simulink model "WorstCaseInertia"  (R2020a)
settings: Solver=VariableStepAuto  StartTime=0.0  StopTime=inf  RelTol=1e-3
libraries: vrlib x7, aerolibanimutils x1, RobotG18_Blocos x1
settings Model: Creator=Catarina  LastModifiedBy=Catarina

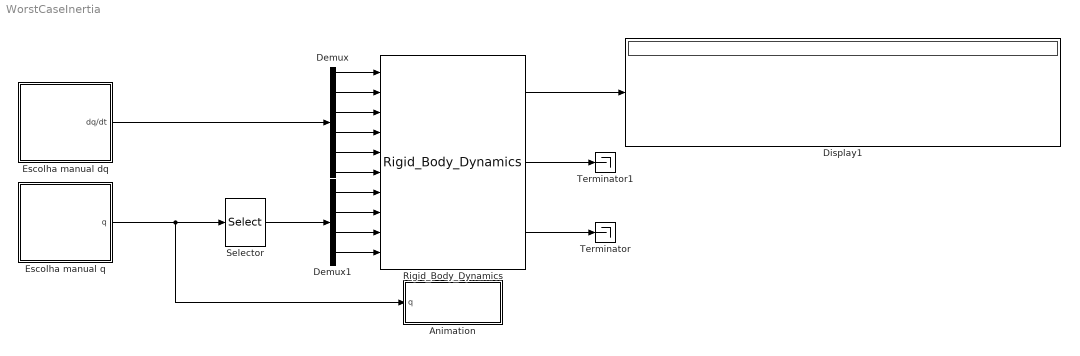
== system WorstCaseInertia ==
  "Animation " : Subsystem
  Demux : Demux  Outputs=6
  Demux1 : Demux
  Display1 : Display
  Escolha manual dq : Subsystem  mask{q1=9.800, q2=-1.400, q3=10.0, q4=-10.0, q5=-5.600, q6=-6.400}
      mask prompts: q1 "dq1"; q2 "dq2"; q3 "dq3"; q4 "dq4"; q5 "dq5"; q6 "dq6"
  "Escolha manual q " : Subsystem  mask{q1=0, q2=0, q3=0, q4=-111, q5=-90.0, q6=0}
  Rigid_Body_Dynamics : RobotG18_Blocos/Rigid_Body_Dynamics  SystemSampleTime=-1  Latency=0  AutoFrameSizeCalculation=off
  Selector : Selector  InputPortWidth=6  IndexOptions=Index vector (dialog)  Indices=[2 3 4 5]  OutputSizes=1
  Terminator : Terminator
  Terminator1 : Terminator
  wires:
  Demux/6 -> Rigid_Body_Dynamics/6
  Demux1/1 -> Rigid_Body_Dynamics/7
  Demux/3 -> Rigid_Body_Dynamics/3
  Demux/5 -> Rigid_Body_Dynamics/5
  Demux/4 -> Rigid_Body_Dynamics/4
  Demux1/2 -> Rigid_Body_Dynamics/8
  Demux/1 -> Rigid_Body_Dynamics/1
  Demux1/3 -> Rigid_Body_Dynamics/9
  Demux1/4 -> Rigid_Body_Dynamics/10
  Demux/2 -> Rigid_Body_Dynamics/2
  "Escolha manual q "/1("q ") -> "Animation "/1("q "), Selector/1
  Escolha manual dq/1("dq/dt ") -> Demux/1
  Selector/1 -> Demux1/1
  Rigid_Body_Dynamics/2 -> Terminator1/1
  Rigid_Body_Dynamics/3 -> Terminator/1
  Rigid_Body_Dynamics/1 -> Display1/1

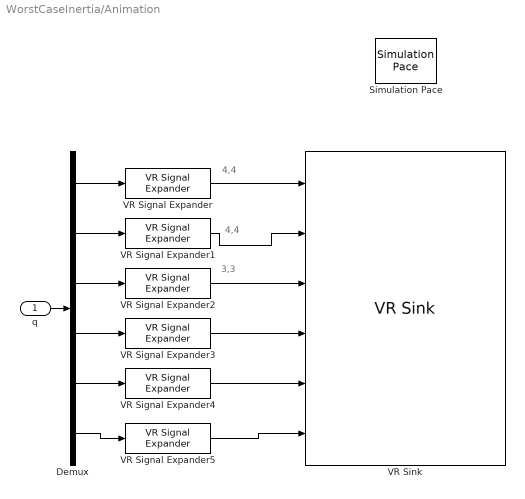
== system WorstCaseInertia/Animation  ==
  note: 4,4
  note: 3,3
  note: 4,4
  "q " : Inport
  Demux : Demux  Outputs=6
  Simulation Pace : aerolibanimutils/Simulation Pace  SimulationPace=1  SleepMode=Auto  OutputPaceError=off  SampleTime=1/30
  VR Signal Expander{,1..5} (6 alike) : vrlib/VR Signal Expander  outwidth=4  outidx=4
  VR Sink : vrlib/VR Sink  InstantiateOnLoad=on  SampleTime=1/30  ViewEnable=on  RemoteChange=off  RemoteView=off  FieldsWritten=Jt1_DH_dv.rotation.4.1.1.double#Jt2_DH_dv.rotation.4.1.1.double#Jt3_DH_dv.rotation.4.1.1.double#Jt4_DH_dv.rotation.4.1.1.double#Jt5_DH_dv.rotation.4.1.1.double#Jt6_DH_dv.rotation.4.1.1.double  WorldFileName=RobotG18_Opt_NoAxes.wrl  WorldDescription=D-H Reference Frames for Virtual Reality Robot  AutoView=off  VideoDimensions=[]  AllowVariableSize=off  FigureProperties="{'Position', 'Name', 'Viewpoint', 'CameraBound', 'CameraDirection', 'CameraPosition', 'CameraUpVector', 'ZoomFactor', 'Antialiasing', 'Headlight', 'Lighting', 'NavPanel', 'Sound', 'StatusBar', 'Stereo3D', 'Stereo3DCameraOffset', 'Stereo3DHIT', 'ToolBar', 'Textures', 'Transparency', 'Triad', 'Wireframe', 'NavZones', 'NavMode', 'NavSpeed', 'CaptureFileFormat', 'CaptureFileName', 'Record2DCompressMethod', 'Record2DCompressQuality', 'Record2D', 'Record2DFileName', 'Record2DFPS'; [3.2740000000000003e+02   1.0300000000000000e+02   5.7600000000000000e+02   3.5000000000000000e+02], 'D-H Reference Frames for Virtual Reality Robot', 'View 1', 'on', [0.0000000000000000e+00  -3.4289780745545140e-01  -9.3937271284737911e-01], [0.0000000000000000e+00   0.0000000000000000e+00   0.0000000000000000e+00], [0.0000000000000000e+00   9.3937271284737911e-01  -3.4289780745545140e-01], [1.0000000000000000e+00], 'on', 'on', 'on', 'halfbar', 'on', 'on', 'off', [1.0000000149011612e-01], [0.0000000000000000e+00], 'on', 'on', 'on', 'none', 'off', 'off', 'examine', 'normal', 'tif', '%f_anim_%n.tif', 'auto', [7.5000000000000000e+01], 'off', '%f_anim_%n.avi', 'auto'}"
  wires:
  "q "/1 -> Demux/1
  Demux/1 -> VR Signal Expander/1
  Demux/2 -> VR Signal Expander1/1
  Demux/3 -> VR Signal Expander2/1
  Demux/4 -> VR Signal Expander3/1
  Demux/5 -> VR Signal Expander4/1
  Demux/6 -> VR Signal Expander5/1
  VR Signal Expander/1 -> VR Sink/1
  VR Signal Expander1/1 -> VR Sink/2
  VR Signal Expander5/1 -> VR Sink/6
  VR Signal Expander2/1 -> VR Sink/3
  VR Signal Expander3/1 -> VR Sink/4
  VR Signal Expander4/1 -> VR Sink/5

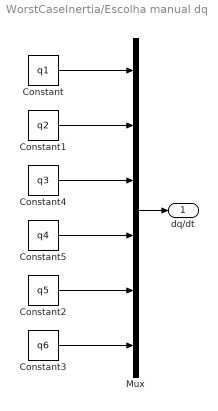
== system WorstCaseInertia/Escolha manual dq ==
  Constant : Constant  Value=q1
  Constant1 : Constant  Value=q2
  Constant2 : Constant  Value=q5
  Constant3 : Constant  Value=q6
  Constant4 : Constant  Value=q3
  Constant5 : Constant  Value=q4
  Mux : Mux  Inputs=6
  "dq/dt " : Outport
  wires:
  Mux/1 -> "dq/dt "/1
  Constant/1 -> Mux/1
  Constant1/1 -> Mux/2
  Constant4/1 -> Mux/3
  Constant5/1 -> Mux/4
  Constant2/1 -> Mux/5
  Constant3/1 -> Mux/6

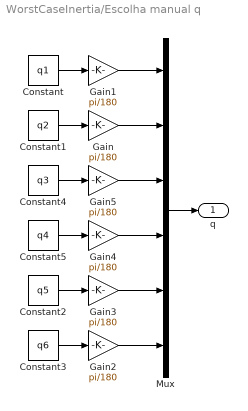
== system WorstCaseInertia/Escolha manual q  ==
  Constant : Constant  Value=q1
  Constant1 : Constant  Value=q2
  Constant2 : Constant  Value=q5
  Constant3 : Constant  Value=q6
  Constant4 : Constant  Value=q3
  Constant5 : Constant  Value=q4
  Gain{,1..5} (6 alike) : Gain  Gain=pi/180
  Mux : Mux  Inputs=6
  "q " : Outport
  wires:
  Constant/1 -> Gain1/1
  Constant1/1 -> Gain/1
  Mux/1 -> "q "/1
  Gain1/1 -> Mux/1
  Gain/1 -> Mux/2
  Constant2/1 -> Gain3/1
  Constant3/1 -> Gain2/1
  Constant4/1 -> Gain5/1
  Constant5/1 -> Gain4/1
  Gain5/1 -> Mux/3
  Gain4/1 -> Mux/4
  Gain3/1 -> Mux/5
  Gain2/1 -> Mux/6
